simulink model "chap10_3"  (Simulink 3.00)
settings: Solver=ode45  StartTime=0.0  StopTime=100  RelTol=1e-3

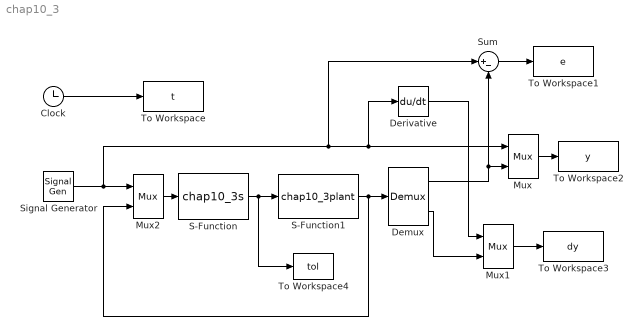
== system chap10_3 ==
  Clock : Clock
      settings: DisplayTime=off  Decimation=10
  Demux : Demux  Outputs=2
  Derivative : Derivative
  Mux : Mux  Inputs=2
      settings: DisplayOption=none
  Mux1 : Mux  Inputs=2
      settings: DisplayOption=none
  Mux2 : Mux  Inputs=2
      settings: DisplayOption=none
  S-Function : S-Function  FunctionName=chap10_3s  PortCounts=[]  SFunctionModules=''
  S-Function1 : S-Function  FunctionName=chap10_3plant  PortCounts=[]  SFunctionModules=''
  Signal Generator : SignalGenerator  WaveForm=sine  Amplitude=2  Frequency=0.1  Units=Hertz
  Sum : Sum  Inputs=|+-  SaturateOnIntegerOverflow=on
  To Workspace : ToWorkspace  VariableName=t  SampleTime=-1  SaveFormat=Matrix
  To Workspace1 : ToWorkspace  VariableName=e  SampleTime=-1  SaveFormat=Matrix
  To Workspace2 : ToWorkspace  VariableName=y  SampleTime=-1  SaveFormat=Matrix
  To Workspace3 : ToWorkspace  VariableName=dy  SampleTime=-1  SaveFormat=Matrix
  To Workspace4 : ToWorkspace  VariableName=tol  SampleTime=-1  SaveFormat=Matrix
  wires:
  Clock/1 -> To Workspace/1
  Sum/1 -> To Workspace1/1
  Mux/1 -> To Workspace2/1
  Demux/1 -> Mux/2, Sum/2
  S-Function1/1 -> Demux/1, Mux2/2
  Mux2/1 -> S-Function/1
  Signal Generator/1 -> Sum/1, Mux/1, Derivative/1, Mux2/1
  Mux1/1 -> To Workspace3/1
  Demux/2 -> Mux1/2
  Derivative/1 -> Mux1/1
  S-Function/1 -> S-Function1/1, To Workspace4/1
